simulink library "dxlSimLibrary"  (R2020a)
settings: Solver=VariableStepAuto  StartTime=0.0  StopTime=10.0  RelTol=1e-3
undefined symbols (not defined in the file): group_num_read, group_num_write, lib_name, motor_IDs, motor_models, port_num, protocol_version, select_sync_read, select_sync_write, start_address_read_indirect, Ts
Description:
  | Dynamixel library for Matlab and Simulink
  | Author: Georgios Andrikopoulos (geoand@kth.se), 2022
  | Mechatronics & Embedded Control Systems Unit, KTH, Stockholm
settings Model: Creator=geoand  LastModifiedBy=mluser

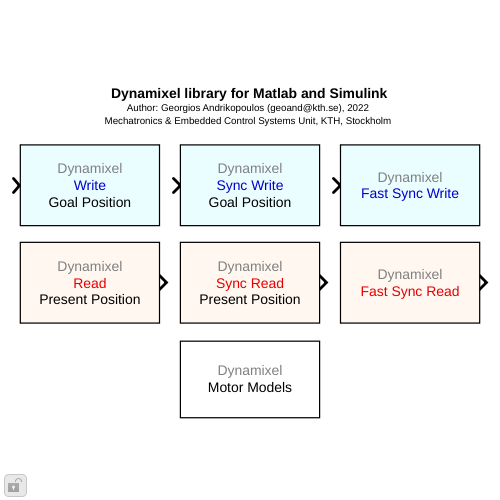
[thumbnail: Simulink's stored preview of the top-level diagram]
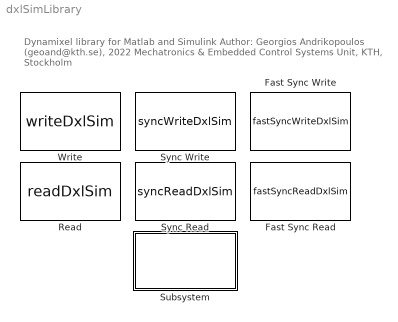
== system dxlSimLibrary ==
  note: Dynamixel library for Matlab and Simulink
      | Author: Georgios Andrikopoulos (geoand@kth.se), 2022
      | Mechatronics & Embedded Control Systems Unit, KTH, Stockholm
  Fast Sync Read : M-S-Function  Description=|  FunctionName=fastSyncReadDxlSim  Parameters=lib_name, group_num_read, ids, models, select_sync_read, start_address_read_indirect, Ts  mask(Dynamixel library for Matlab and Simulink){lib_name=lib_name, group_num_read=group_num_read, ids=motor_IDs, models=motor_models, select_sync_read=select_sync_read, start_address_read_indirect=start_address_read_indirect, Ts=Ts}
      | Dynamixel library for Matlab and Simulink
      | Fast Sync Read function
      | Author: Georgios Andrikopoulos (geoand@kth.se), 2022 
      | Mechatronics & Embedded Control Systems Unit, KTH, Stockholm
      mask prompts: lib_name "Library Name"; group_num_read "Group Number"; ids "Motor IDs"; models "Motor models"; select_sync_read "Sync Read Selection"; start_address_read_indirect "Start Address (Indirect)"; Ts "Sampling Time"
      mask help:
      | Library block for execution of sync read for 1 or more Dynamixel motors in Simulink
      |
      | Part of the Dynamixel library for Matlab and Simulink
      | Author: Georgios Andrikopoulos (geoand@kth.se), 2022
      | Mechatronics & Embedded Control Systems Unit, KTH, Stockholm
      mask Help:
      | Library block for execution of sync read for 1 or more Dynamixel motors in Simulink
      | 
      | Part of the Dynamixel library for Matlab and Simulink
      | Author: Georgios Andrikopoulos (geoand@kth.se), 2022
      | Mechatronics & Embedded Control Systems Unit, KTH, Stockholm
      mask Display:
      | color('gray')
      | fprintf('\nDynamixel\n\n');
      | color('red')
      | fprintf('\n\n\nFast Sync Read\n\n');
  Fast Sync Write : M-S-Function  Description=|  FunctionName=fastSyncWriteDxlSim  Parameters=lib_name, group_num_write, ids, models, select_sync_write, Ts  mask(Dynamixel library for Matlab and Simulink){lib_name=lib_name, group_num_write=group_num_write, ids=motor_IDs, models=motor_models, select_sync_write=select_sync_write, Ts=Ts}
      | Dynamixel library for Matlab and Simulink
      | Fast Sync Write function
      | Author: Georgios Andrikopoulos (geoand@kth.se), 2022 
      | Mechatronics & Embedded Control Systems Unit, KTH, Stockholm
      mask prompts: lib_name "Library Name"; group_num_write "Group Number"; ids "Motor IDs"; models "Motor models"; select_sync_write "Sync Write Parameters"; Ts "Samping Time"
      mask help:
      | Library block for execution of sync write for 1 or more Dynamixel motors in Simulink
      |
      | Part of the Dynamixel library for Matlab and Simulink
      | Author: Georgios Andrikopoulos (geoand@kth.se), 2022
      | Mechatronics & Embedded Control Systems Unit, KTH, Stockholm
      mask Help:
      | Library block for execution of sync write for 1 or more Dynamixel motors in Simulink
      | 
      | Part of the Dynamixel library for Matlab and Simulink
      | Author: Georgios Andrikopoulos (geoand@kth.se), 2022
      | Mechatronics & Embedded Control Systems Unit, KTH, Stockholm
      mask Display:
      | color('gray')
      | fprintf('\nDynamixel\n\n');
      | color('blue')
      | fprintf('\n\n\nFast Sync Write\n\n');
  Read : M-S-Function  Description=|  FunctionName=readDxlSim  Parameters=lib_name, port_num, protocol_version, ids, models, select, Ts  mask(Dynamixel Library for MATLAB and Simulink){lib_name=lib_name, port_num=port_num, protocol_version=protocol_version, ids=motor_IDs, models=motor_models, select=Present Position, Ts=Ts}
      | Dynamixel library for Matlab and Simulink
      | Read function
      | Author: Georgios Andrikopoulos (geoand@kth.se), 2022 
      | Mechatronics & Embedded Control Systems Unit, KTH, Stockholm
      mask prompts: lib_name "Library name"; port_num "Port number"; protocol_version "Protocol version"; ids "Motor IDs"; models "Motor models"; select "Read function"; Ts "Sampling time"
      mask help:
      | Library block executing the read() function for 1 or more Dynamixel motors
      | Part of the Dynamixel library for Matlab and Simulink
      | Author: Georgios Andrikopoulos (geoand@kth.se), 2022
      | Mechatronics & Embedded Control Systems Unit, KTH, Stockholm
      mask Help:
      | Library block executing the read() function for 1 or more Dynamixel motors
      | Part of the Dynamixel library for Matlab and Simulink
      | Author: Georgios Andrikopoulos (geoand@kth.se), 2022
      | Mechatronics & Embedded Control Systems Unit, KTH, Stockholm
      mask Display:
      | color('gray')
      | fprintf('Dynamixel\n\n');
      | color('red')
      | fprintf('\n\nRead\n\n');
      | color('black')
      | fprintf('\n\n%s',select);
  Subsystem : Subsystem  Description=|
      | Dynamixel library for Matlab and Simulink
      | Motor Models
      | Author: Georgios Andrikopoulos (geoand@kth.se), 2022 
      | Mechatronics & Embedded Control Systems Unit, KTH, Stockholm
      mask Display:
      | color('gray')
      | fprintf('Dynamixel\n');
      | color('black')
      | fprintf('\nMotor Models');
  Sync Read : M-S-Function  Description=|  FunctionName=syncReadDxlSim  Parameters=lib_name, group_num, ids, models, select, Ts  mask(Dynamixel Library for MATLAB and Simulink){lib_name=lib_name, group_num=group_num_read(1), ids=motor_IDs, models=motor_models, select=Present Position, Ts=Ts}
      | Dynamixel library for Matlab and Simulink
      | Sync Read function
      | Author: Georgios Andrikopoulos (geoand@kth.se), 2022 
      | Mechatronics & Embedded Control Systems Unit, KTH, Stockholm
      mask prompts: lib_name "Library name"; group_num "Group number"; ids "Motor IDs"; models "Motor models"; select "Read function"; Ts "Sampling time"
      mask help:
      | Library block executing the syncread() function for 1 or more Dynamixel motors
      | Part of the Dynamixel library for Matlab and Simulink
      | Author: Georgios Andrikopoulos (geoand@kth.se), 2022
      | Mechatronics & Embedded Control Systems Unit, KTH, Stockholm
      mask Help:
      | Library block executing the syncread() function for 1 or more Dynamixel motors
      | Part of the Dynamixel library for Matlab and Simulink
      | Author: Georgios Andrikopoulos (geoand@kth.se), 2022
      | Mechatronics & Embedded Control Systems Unit, KTH, Stockholm
      mask Display:
      | color('gray')
      | fprintf('Dynamixel\n\n');
      | color('red')
      | fprintf('\n\nSync Read\n\n');
      | color('black')
      | fprintf('\n\n%s',select);
  Sync Write : M-S-Function  Description=|  FunctionName=syncWriteDxlSim  Parameters=lib_name, group_num, ids, models, select, Ts  mask(Dynamixel Library for MATLAB and Simulink){lib_name=lib_name, group_num=group_num_write(1), ids=motor_IDs, models=motor_models, select=Goal Position, Ts=Ts}
      | Dynamixel library for Matlab and Simulink
      | Sync Write function
      | Author: Georgios Andrikopoulos (geoand@kth.se), 2022 
      | Mechatronics & Embedded Control Systems Unit, KTH, Stockholm
      mask prompts: lib_name "Library name"; group_num "Group number"; ids "Motor IDs"; models "Motor models"; select "Write function"; Ts "Sampling time"
      mask help:
      | Library block executing the syncwrite() function for 1 or more Dynamixel motors
      | Part of the Dynamixel library for Matlab and Simulink
      | Author: Georgios Andrikopoulos (geoand@kth.se), 2022
      | Mechatronics & Embedded Control Systems Unit, KTH, Stockholm
      mask Help:
      | Library block executing the syncwrite() function for 1 or more Dynamixel motors
      | Part of the Dynamixel library for Matlab and Simulink
      | Author: Georgios Andrikopoulos (geoand@kth.se), 2022
      | Mechatronics & Embedded Control Systems Unit, KTH, Stockholm
      mask Display:
      | color('gray')
      | fprintf('Dynamixel\n\n');
      | color('blue')
      | fprintf('\n\nSync Write\n\n');
      | color('black')
      | fprintf('\n\n%s',select);
  Write : M-S-Function  Description=|  FunctionName=writeDxlSim  Parameters=lib_name, port_num, protocol_version, ids, models, select, Ts  mask(Dynamixel Library for MATLAB and Simulink){lib_name=lib_name, port_num=port_num, protocol_version=protocol_version, ids=motor_IDs, models=motor_models, select=Goal Position, Ts=Ts}
      | Dynamixel library for Matlab and Simulink
      | Write function
      | Author: Georgios Andrikopoulos (geoand@kth.se), 2022 
      | Mechatronics & Embedded Control Systems Unit, KTH, Stockholm
      mask prompts: lib_name "Library name"; port_num "Port number"; protocol_version "Protocol version"; ids "Motor IDs"; models "Motor models"; select "Write function"; Ts "Sampling time"
      mask help:
      | Library block executing the write() function for 1 or more Dynamixel motors
      | Part of the Dynamixel library for Matlab and Simulink
      | Author: Georgios Andrikopoulos (geoand@kth.se), 2022
      | Mechatronics & Embedded Control Systems Unit, KTH, Stockholm
      mask Help:
      | Library block executing the write() function for 1 or more Dynamixel motors
      | Part of the Dynamixel library for Matlab and Simulink
      | Author: Georgios Andrikopoulos (geoand@kth.se), 2022
      | Mechatronics & Embedded Control Systems Unit, KTH, Stockholm
      mask Display:
      | color('gray')
      | fprintf('Dynamixel\n\n');
      | color('blue')
      | fprintf('\n\nWrite\n\n');
      | color('black')
      | fprintf('\n\n%s',select);

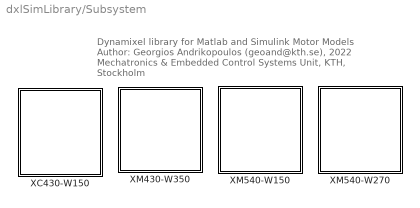
== system dxlSimLibrary/Subsystem ==
  note: Dynamixel library for Matlab and Simulink
      | Motor Models
      | Author: Georgios Andrikopoulos (geoand@kth.se), 2022
      | Mechatronics & Embedded Control Systems Unit, KTH, Stockholm
  XC430-W150 : Subsystem  Description=|
      | Dynamixel library for Matlab and Simulink
      | Motor Models
      | Author: Georgios Andrikopoulos (geoand@kth.se), 2022 
      | Mechatronics & Embedded Control Systems Unit, KTH, Stockholm
      mask Display: image('$imagefile'); % Use "Edit Image" on toolstrip to change.
  "XM430-W350 " : Subsystem  Description=|
      | Dynamixel library for Matlab and Simulink
      | Motor Models
      | Author: Georgios Andrikopoulos (geoand@kth.se), 2022 
      | Mechatronics & Embedded Control Systems Unit, KTH, Stockholm
      mask Display: image('$imagefile'); % Use "Edit Image" on toolstrip to change.
  XM540-W150 : Subsystem  Description=|
      | Dynamixel library for Matlab and Simulink
      | Motor Models
      | Author: Georgios Andrikopoulos (geoand@kth.se), 2022 
      | Mechatronics & Embedded Control Systems Unit, KTH, Stockholm
      mask Display: image('$imagefile'); % Use "Edit Image" on toolstrip to change.
  XM540-W270 : Subsystem  Description=|
      | Dynamixel library for Matlab and Simulink
      | Motor Models
      | Author: Georgios Andrikopoulos (geoand@kth.se), 2022 
      | Mechatronics & Embedded Control Systems Unit, KTH, Stockholm
      mask Display: image('$imagefile'); % Use "Edit Image" on toolstrip to change.

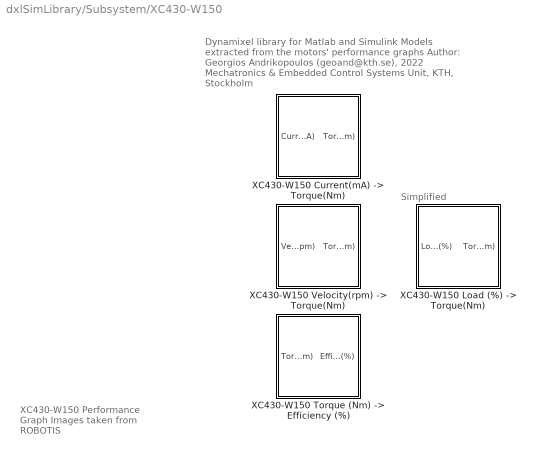
== system dxlSimLibrary/Subsystem/XC430-W150 ==
  note: Simplified
  note: Dynamixel library for Matlab and Simulink
      | Models extracted from the motors' performance graphs
      | Author: Georgios Andrikopoulos (geoand@kth.se), 2022
      | Mechatronics & Embedded Control Systems Unit, KTH, Stockholm
  note: XC430-W150 Performance Graph
      | Images taken from ROBOTIS
  "XC430-W150 Current(mA) -> Torque(Nm)" : Subsystem  Description=|
      | Dynamixel library for Matlab and Simulink
      | Author: Georgios Andrikopoulos (geoand@kth.se), 2022 
      | Mechatronics & Embedded Control Systems Unit, KTH, Stockholm
      mask Display: image('$imagefile'); % Use "Edit Image" on toolstrip to change.
  "XC430-W150 Load (%) -> Torque(Nm)" : Subsystem  Description=|
      | Dynamixel library for Matlab and Simulink
      | Author: Georgios Andrikopoulos (geoand@kth.se), 2022 
      | Mechatronics & Embedded Control Systems Unit, KTH, Stockholm
      mask Display: image('$imagefile'); % Use "Edit Image" on toolstrip to change.
  "XC430-W150 Torque (Nm) -> Efficiency (%)" : Subsystem  Description=|
      | Dynamixel library for Matlab and Simulink
      | Author: Georgios Andrikopoulos (geoand@kth.se), 2022 
      | Mechatronics & Embedded Control Systems Unit, KTH, Stockholm
      mask Display: image('$imagefile'); % Use "Edit Image" on toolstrip to change.
  "XC430-W150 Velocity(rpm) -> Torque(Nm)" : Subsystem  Description=|
      | Dynamixel library for Matlab and Simulink
      | Author: Georgios Andrikopoulos (geoand@kth.se), 2022 
      | Mechatronics & Embedded Control Systems Unit, KTH, Stockholm
      mask Display: image('$imagefile'); % Use "Edit Image" on toolstrip to change.

== system dxlSimLibrary/Subsystem/XM430-W350  ==
  note: Dynamixel library for Matlab and Simulink
      | Models extracted from the motors' performance graphs
      | Author: Georgios Andrikopoulos (geoand@kth.se), 2022
      | Mechatronics & Embedded Control Systems Unit, KTH, Stockholm
  note: XM430-W350 Performance Graph
      | Images taken from ROBOTIS
  "XM430-W350 Current(mA) -> Torque(Nm)" : Subsystem  Description=|
      | Dynamixel library for Matlab and Simulink
      | Author: Georgios Andrikopoulos (geoand@kth.se), 2022 
      | Mechatronics & Embedded Control Systems Unit, KTH, Stockholm
      mask Display: image('$imagefile'); % Use "Edit Image" on toolstrip to change.
  "XM430-W350 Torque (Nm) -> Efficiency (%)" : Subsystem  Description=|
      | Dynamixel library for Matlab and Simulink
      | Author: Georgios Andrikopoulos (geoand@kth.se), 2022 
      | Mechatronics & Embedded Control Systems Unit, KTH, Stockholm
      mask Display: image('$imagefile'); % Use "Edit Image" on toolstrip to change.
  "XM430-W350 Velocity(rpm) -> Torque(Nm)" : Subsystem  Description=|
      | Dynamixel library for Matlab and Simulink
      | Author: Georgios Andrikopoulos (geoand@kth.se), 2022 
      | Mechatronics & Embedded Control Systems Unit, KTH, Stockholm
      mask Display: image('$imagefile'); % Use "Edit Image" on toolstrip to change.

== system dxlSimLibrary/Subsystem/XM540-W150 ==
  note: Dynamixel library for Matlab and Simulink
      | Models extracted from the motors' performance graphs
      | Author: Georgios Andrikopoulos (geoand@kth.se), 2022
      | Mechatronics & Embedded Control Systems Unit, KTH, Stockholm
  note: XM540-W150 Performance Graph
      | Images taken from ROBOTIS
  "XM540-W150 Current(mA) -> Torque(Nm)" : Subsystem  Description=|
      | Dynamixel library for Matlab and Simulink
      | Author: Georgios Andrikopoulos (geoand@kth.se), 2022 
      | Mechatronics & Embedded Control Systems Unit, KTH, Stockholm
      mask Display: image('$imagefile'); % Use "Edit Image" on toolstrip to change.
  "XM540-W150 Torque (Nm) -> Efficiency (%)" : Subsystem  Description=|
      | Dynamixel library for Matlab and Simulink
      | Author: Georgios Andrikopoulos (geoand@kth.se), 2022 
      | Mechatronics & Embedded Control Systems Unit, KTH, Stockholm
      mask Display: image('$imagefile'); % Use "Edit Image" on toolstrip to change.
  "XM540-W150 Velocity(rpm) -> Torque(Nm)" : Subsystem  Description=|
      | Dynamixel library for Matlab and Simulink
      | Author: Georgios Andrikopoulos (geoand@kth.se), 2022 
      | Mechatronics & Embedded Control Systems Unit, KTH, Stockholm
      mask Display: image('$imagefile'); % Use "Edit Image" on toolstrip to change.

== system dxlSimLibrary/Subsystem/XM540-W270 ==
  note: Dynamixel library for Matlab and Simulink
      | Models extracted from the motors' performance graphs
      | Author: Georgios Andrikopoulos (geoand@kth.se), 2022
      | Mechatronics & Embedded Control Systems Unit, KTH, Stockholm
  note: XM540-W270 Performance Graph
      | Images taken from ROBOTIS
  "XM540-W270 Current(mA) -> Torque(Nm)" : Subsystem  Description=|
      | Dynamixel library for Matlab and Simulink
      | Author: Georgios Andrikopoulos (geoand@kth.se), 2022 
      | Mechatronics & Embedded Control Systems Unit, KTH, Stockholm
      mask Display: image('$imagefile'); % Use "Edit Image" on toolstrip to change.
  "XM540-W270 Torque (Nm) -> Efficiency (%)" : Subsystem  Description=|
      | Dynamixel library for Matlab and Simulink
      | Author: Georgios Andrikopoulos (geoand@kth.se), 2022 
      | Mechatronics & Embedded Control Systems Unit, KTH, Stockholm
      mask Display: image('$imagefile'); % Use "Edit Image" on toolstrip to change.
  "XM540-W270 Velocity(rpm) -> Torque(Nm)" : Subsystem  Description=|
      | Dynamixel library for Matlab and Simulink
      | Author: Georgios Andrikopoulos (geoand@kth.se), 2022 
      | Mechatronics & Embedded Control Systems Unit, KTH, Stockholm
      mask Display: image('$imagefile'); % Use "Edit Image" on toolstrip to change.

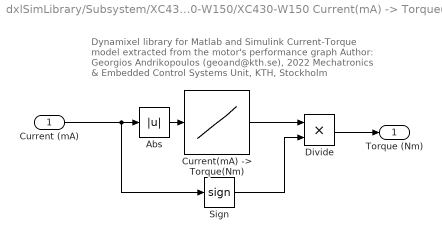
== system dxlSimLibrary/Subsystem/XC430-W150/XC430-W150 Current(mA) -> Torque(Nm) ==
  note: Dynamixel library for Matlab and Simulink
      | Current-Torque model extracted from the motor's performance graph
      | Author: Georgios Andrikopoulos (geoand@kth.se), 2022
      | Mechatronics & Embedded Control Systems Unit, KTH, Stockholm
  Current (mA) : Inport
  Abs : Abs
  "Current(mA) -> Torque(Nm)" : Lookup_n-D  NumberOfTableDimensions=1  BreakpointsForDimension1="[0 200    218    334    458    602    766    952    1164    1270]"  BreakpointsForDimension1DataTypeStr=double  Table="[0 0.0890    0.1030    0.2000    0.3000    0.4000    0.5000    0.6000    0.7000    0.7420]"  TableDataTypeStr=double  IntermediateResultsDataTypeStr=double  InternalRulePriority=Speed  OutDataTypeStr=double  RndMeth=Simplest  FractionDataTypeStr=double
  Divide : Product  Inputs=**
  Sign : Signum
  Torque (Nm) : Outport
  wires:
  Abs/1 -> "Current(mA) -> Torque(Nm)"/1
  "Current(mA) -> Torque(Nm)"/1 -> Divide/1
  Divide/1 -> Torque (Nm)/1
  Sign/1 -> Divide/2
  Current (mA)/1 -> Sign/1, Abs/1

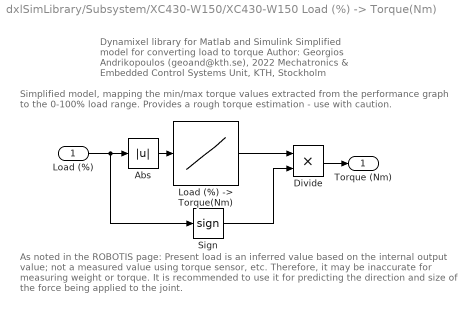
== system dxlSimLibrary/Subsystem/XC430-W150/XC430-W150 Load (%) -> Torque(Nm) ==
  note: As noted in the ROBOTIS page:
      | Present load is an inferred value based on the internal output value; not a measured value using torque sensor, etc. Therefore, it may be inaccurate for measuring weight or torque. It is recommended to use it for predicting the direction and size of the force being applied to the joint.
  note: Simplified model, mapping the min/max torque values extracted from the performance graph to the 0-100% load range. Provides a rough torque estimation - use with caution.
  note: Dynamixel library for Matlab and Simulink
      | Simplified model for converting load to torque
      | Author: Georgios Andrikopoulos (geoand@kth.se), 2022
      | Mechatronics & Embedded Control Systems Unit, KTH, Stockholm
  Load (%) : Inport
  Abs : Abs
  Divide : Product  Inputs=**
  "Load (%) -> Torque(Nm)" : Lookup_n-D  NumberOfTableDimensions=1  BreakpointsForDimension1=[0 100]  BreakpointsForDimension1DataTypeStr=double  Table=[0.0890 0.7420]  TableDataTypeStr=double  IntermediateResultsDataTypeStr=double  InternalRulePriority=Speed  OutDataTypeStr=double  RndMeth=Simplest  FractionDataTypeStr=double
  Sign : Signum
  Torque (Nm) : Outport
  wires:
  Load (%)/1 -> Sign/1, Abs/1
  "Load (%) -> Torque(Nm)"/1 -> Divide/1
  Abs/1 -> "Load (%) -> Torque(Nm)"/1
  Sign/1 -> Divide/2
  Divide/1 -> Torque (Nm)/1

== system dxlSimLibrary/Subsystem/XC430-W150/XC430-W150 Torque (Nm) -> Efficiency (%) ==
  note: Dynamixel library for Matlab and Simulink
      | Torque-Efficiency model extracted from the motor's performance graph
      | Author: Georgios Andrikopoulos (geoand@kth.se), 2022
      | Mechatronics & Embedded Control Systems Unit, KTH, Stockholm
  Torque (Nm) : Inport
  Abs1 : Abs
  "Torque (Nm) -> Efficiency (%)" : Lookup_n-D  NumberOfTableDimensions=1  BreakpointsForDimension1="[0.0890    0.1030    0.2000    0.3000    0.4000    0.5000    0.6000    0.7000    0.7420]"  BreakpointsForDimension1DataTypeStr=Inherit: Inherit from 'Breakpoint data'  Table="[36.7000   40.0000   46.1000   43.3000   37.9000   31.0000   21.6000   10.5000    5.2000]"  InternalRulePriority=Speed  RndMeth=Simplest  InputSameDT=on
  Efficiency (%) : Outport
  wires:
  "Torque (Nm) -> Efficiency (%)"/1 -> Efficiency (%)/1
  Abs1/1 -> "Torque (Nm) -> Efficiency (%)"/1
  Torque (Nm)/1 -> Abs1/1

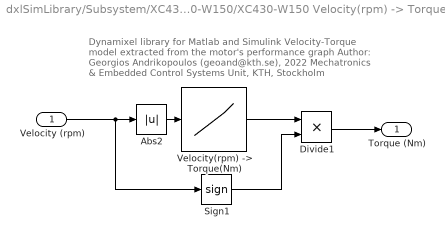
== system dxlSimLibrary/Subsystem/XC430-W150/XC430-W150 Velocity(rpm) -> Torque(Nm) ==
  note: Dynamixel library for Matlab and Simulink
      | Velocity-Torque model extracted from the motor's performance graph
      | Author: Georgios Andrikopoulos (geoand@kth.se), 2022
      | Mechatronics & Embedded Control Systems Unit, KTH, Stockholm
  Velocity (rpm) : Inport
  Abs2 : Abs
  Divide1 : Product  Inputs=**
  Sign1 : Signum
  "Velocity(rpm) -> Torque(Nm)" : Lookup_n-D  NumberOfTableDimensions=1  BreakpointsForDimension1="[7.7000   18.0400   37.4000   53.4600   67.1000   78.9800   89.4300   98.7800  100.2100]"  BreakpointsForDimension1DataTypeStr=double  Table="[0.7420    0.7000    0.6000    0.5000    0.4000    0.3000    0.2000    0.1030    0.0890]"  TableDataTypeStr=double  IntermediateResultsDataTypeStr=double  InternalRulePriority=Speed  OutDataTypeStr=double  RndMeth=Simplest  FractionDataTypeStr=double  InputSameDT=on
  Torque (Nm) : Outport
  wires:
  Divide1/1 -> Torque (Nm)/1
  Velocity (rpm)/1 -> Sign1/1, Abs2/1
  Sign1/1 -> Divide1/2
  Abs2/1 -> "Velocity(rpm) -> Torque(Nm)"/1
  "Velocity(rpm) -> Torque(Nm)"/1 -> Divide1/1

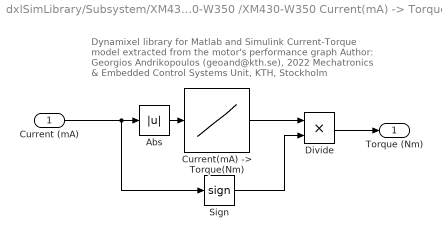
== system dxlSimLibrary/Subsystem/XM430-W350 /XM430-W350 Current(mA) -> Torque(Nm) ==
  note: Dynamixel library for Matlab and Simulink
      | Current-Torque model extracted from the motor's performance graph
      | Author: Georgios Andrikopoulos (geoand@kth.se), 2022
      | Mechatronics & Embedded Control Systems Unit, KTH, Stockholm
  Current (mA) : Inport
  Abs : Abs
  "Current(mA) -> Torque(Nm)" : Lookup_n-D  NumberOfTableDimensions=1  BreakpointsForDimension1=|  BreakpointsForDimension1DataTypeStr=double  Table=|  TableDataTypeStr=double  IntermediateResultsDataTypeStr=double  InternalRulePriority=Speed  OutDataTypeStr=double  RndMeth=Simplest  FractionDataTypeStr=double
      BreakpointsForDimension1=|
      | [0; 114
      | 270
      | 471
      | 672
      | 867
      | 1080
      | 1275
      | 1485
      | 1692
      | 1797]
      Table=|
      | [0; 0.056
      | 0.350
      | 0.700
      | 1.050
      | 1.400
      | 1.750
      | 2.100
      | 2.450
      | 2.800
      | 3.010]
  Divide : Product  Inputs=**
  Sign : Signum
  Torque (Nm) : Outport
  wires:
  Abs/1 -> "Current(mA) -> Torque(Nm)"/1
  "Current(mA) -> Torque(Nm)"/1 -> Divide/1
  Divide/1 -> Torque (Nm)/1
  Sign/1 -> Divide/2
  Current (mA)/1 -> Sign/1, Abs/1

== system dxlSimLibrary/Subsystem/XM430-W350 /XM430-W350 Torque (Nm) -> Efficiency (%) ==
  note: Dynamixel library for Matlab and Simulink
      | Torque-Efficiency model extracted from the motor's performance graph
      | Author: Georgios Andrikopoulos (geoand@kth.se), 2022
      | Mechatronics & Embedded Control Systems Unit, KTH, Stockholm
  Current (mA) : Inport
  Abs1 : Abs
  "Torque (Nm) -> Efficiency (%)" : Lookup_n-D  NumberOfTableDimensions=1  BreakpointsForDimension1=[0.056,0.350,0.700,1.050,1.400,1.750,2.100,2.450,2.800,3.010]  BreakpointsForDimension1DataTypeStr=Inherit: Inherit from 'Breakpoint data'  Table=[12.70,35,43.50,44.30,41.20,36,29.70,22.40,14.50,9.70]  InternalRulePriority=Speed  RndMeth=Simplest  InputSameDT=on
  Torque (Nm) : Outport
  wires:
  Abs1/1 -> "Torque (Nm) -> Efficiency (%)"/1
  "Torque (Nm) -> Efficiency (%)"/1 -> Torque (Nm)/1
  Current (mA)/1 -> Abs1/1

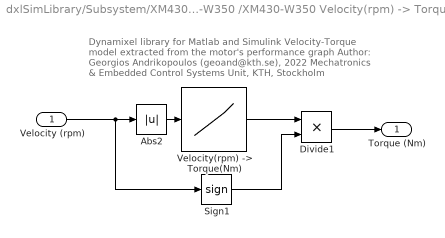
== system dxlSimLibrary/Subsystem/XM430-W350 /XM430-W350 Velocity(rpm) -> Torque(Nm) ==
  note: Dynamixel library for Matlab and Simulink
      | Velocity-Torque model extracted from the motor's performance graph
      | Author: Georgios Andrikopoulos (geoand@kth.se), 2022
      | Mechatronics & Embedded Control Systems Unit, KTH, Stockholm
  Velocity (rpm) : Inport
  Abs2 : Abs
  Divide1 : Product  Inputs=**
  Sign1 : Signum
  "Velocity(rpm) -> Torque(Nm)" : Lookup_n-D  NumberOfTableDimensions=1  BreakpointsForDimension1=[7.76,10.32,14.96,19.60,24,28.56,33.04,37.68,42.08,46.08]  BreakpointsForDimension1DataTypeStr=double  Table=[3.010,2.800,2.450,2.100,1.750,1.400,1.050,0.700,0.350,0.056]  TableDataTypeStr=double  IntermediateResultsDataTypeStr=double  InternalRulePriority=Speed  OutDataTypeStr=double  RndMeth=Simplest  FractionDataTypeStr=double  InputSameDT=on
  Torque (Nm) : Outport
  wires:
  Sign1/1 -> Divide1/2
  Divide1/1 -> Torque (Nm)/1
  Velocity (rpm)/1 -> Sign1/1, Abs2/1
  "Velocity(rpm) -> Torque(Nm)"/1 -> Divide1/1
  Abs2/1 -> "Velocity(rpm) -> Torque(Nm)"/1

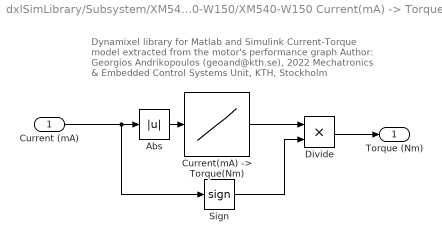
== system dxlSimLibrary/Subsystem/XM540-W150/XM540-W150 Current(mA) -> Torque(Nm) ==
  note: Dynamixel library for Matlab and Simulink
      | Current-Torque model extracted from the motor's performance graph
      | Author: Georgios Andrikopoulos (geoand@kth.se), 2022
      | Mechatronics & Embedded Control Systems Unit, KTH, Stockholm
  Current (mA) : Inport
  Abs : Abs
  "Current(mA) -> Torque(Nm)" : Lookup_n-D  NumberOfTableDimensions=1  BreakpointsForDimension1=|  BreakpointsForDimension1DataTypeStr=double  Table=[0 0.4 0.5 1 1.5 2 2.5 3 3.5 4 4.5]  TableDataTypeStr=double  IntermediateResultsDataTypeStr=double  InternalRulePriority=Speed  OutDataTypeStr=double  RndMeth=Simplest  FractionDataTypeStr=double
      | [0 546
      | 623
      | 1050
      | 1477
      | 1953
      | 2429
      | 2933
      | 3486
      | 4067
      | 4683]
  Divide : Product  Inputs=**
  Sign : Signum
  Torque (Nm) : Outport
  wires:
  Abs/1 -> "Current(mA) -> Torque(Nm)"/1
  "Current(mA) -> Torque(Nm)"/1 -> Divide/1
  Divide/1 -> Torque (Nm)/1
  Sign/1 -> Divide/2
  Current (mA)/1 -> Sign/1, Abs/1

== system dxlSimLibrary/Subsystem/XM540-W150/XM540-W150 Torque (Nm) -> Efficiency (%) ==
  note: Dynamixel library for Matlab and Simulink
      | Torque-Efficiency model extracted from the motor's performance graph
      | Author: Georgios Andrikopoulos (geoand@kth.se), 2022
      | Mechatronics & Embedded Control Systems Unit, KTH, Stockholm
  Current (mA) : Inport
  Abs1 : Abs
  "Torque (Nm) -> Efficiency (%)" : Lookup_n-D  NumberOfTableDimensions=1  BreakpointsForDimension1=[0.4 0.5 1 1.5 2 2.5 3 3.5 4 4.5]  BreakpointsForDimension1DataTypeStr=Inherit: Inherit from 'Breakpoint data'  Table=|  InternalRulePriority=Speed  RndMeth=Simplest  InputSameDT=on
      | [   34.9000
      |    40.0000
      |    49.5000
      |    49.7000
      |    44.8000
      |    38.2000
      |    30.4000
      |    22.0000
      |    13.1000
      |     3.8000]
  Torque (Nm) : Outport
  wires:
  Abs1/1 -> "Torque (Nm) -> Efficiency (%)"/1
  "Torque (Nm) -> Efficiency (%)"/1 -> Torque (Nm)/1
  Current (mA)/1 -> Abs1/1

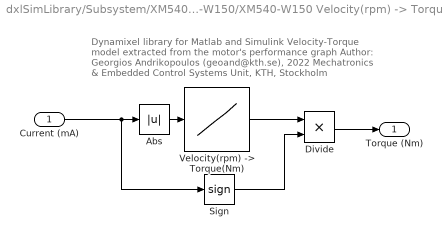
== system dxlSimLibrary/Subsystem/XM540-W150/XM540-W150 Velocity(rpm) -> Torque(Nm) ==
  note: Dynamixel library for Matlab and Simulink
      | Velocity-Torque model extracted from the motor's performance graph
      | Author: Georgios Andrikopoulos (geoand@kth.se), 2022
      | Mechatronics & Embedded Control Systems Unit, KTH, Stockholm
  Current (mA) : Inport
  Abs : Abs
  Divide : Product  Inputs=**
  Sign : Signum
  "Velocity(rpm) -> Torque(Nm)" : Lookup_n-D  NumberOfTableDimensions=1  BreakpointsForDimension1=|  BreakpointsForDimension1DataTypeStr=double  Table=[4.5 4 3.5 3 2.5 2 1.5 1 0.5 0.4]  TableDataTypeStr=double  IntermediateResultsDataTypeStr=double  InternalRulePriority=Speed  OutDataTypeStr=double  RndMeth=Simplest  FractionDataTypeStr=double  InputSameDT=on
      | [    4.4800
      |    13.3700
      |    21.5600
      |    29.4700
      |    36.6800
      |    43.5400
      |    50.4000
      |    56.7000
      |    63.0000
      |    64.1200]
  Torque (Nm) : Outport
  wires:
  Abs/1 -> "Velocity(rpm) -> Torque(Nm)"/1
  "Velocity(rpm) -> Torque(Nm)"/1 -> Divide/1
  Divide/1 -> Torque (Nm)/1
  Sign/1 -> Divide/2
  Current (mA)/1 -> Sign/1, Abs/1

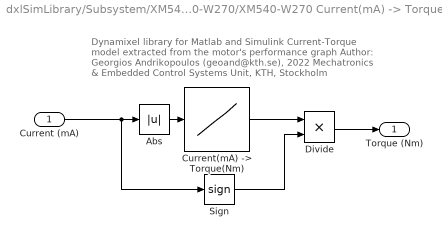
== system dxlSimLibrary/Subsystem/XM540-W270/XM540-W270 Current(mA) -> Torque(Nm) ==
  note: Dynamixel library for Matlab and Simulink
      | Current-Torque model extracted from the motor's performance graph
      | Author: Georgios Andrikopoulos (geoand@kth.se), 2022
      | Mechatronics & Embedded Control Systems Unit, KTH, Stockholm
  Current (mA) : Inport
  Abs : Abs
  "Current(mA) -> Torque(Nm)" : Lookup_n-D  NumberOfTableDimensions=1  BreakpointsForDimension1=|  BreakpointsForDimension1DataTypeStr=double  Table=|  TableDataTypeStr=double  IntermediateResultsDataTypeStr=double  InternalRulePriority=Speed  OutDataTypeStr=double  RndMeth=Simplest  FractionDataTypeStr=double
      BreakpointsForDimension1=|
      | [0; 301
      | 497
      | 847
      | 1246
      | 1659
      | 2114
      | 2597
      | 3129
      | 3703
      | 4060]
      Table=|
      | [0; 0.4
      | 1
      | 2
      | 3
      | 4
      | 5
      | 6
      | 7
      | 8
      | 8.6]
  Divide : Product  Inputs=**
  Sign : Signum
  Torque (Nm) : Outport
  wires:
  Abs/1 -> "Current(mA) -> Torque(Nm)"/1
  "Current(mA) -> Torque(Nm)"/1 -> Divide/1
  Divide/1 -> Torque (Nm)/1
  Sign/1 -> Divide/2
  Current (mA)/1 -> Sign/1, Abs/1

== system dxlSimLibrary/Subsystem/XM540-W270/XM540-W270 Torque (Nm) -> Efficiency (%) ==
  note: Dynamixel library for Matlab and Simulink
      | Torque-Efficiency model extracted from the motor's performance graph
      | Author: Georgios Andrikopoulos (geoand@kth.se), 2022
      | Mechatronics & Embedded Control Systems Unit, KTH, Stockholm
  Current (mA) : Inport
  Abs1 : Abs
  "Torque(Nm) -> Efficiency(%)" : Lookup_n-D  NumberOfTableDimensions=1  BreakpointsForDimension1=|  BreakpointsForDimension1DataTypeStr=Inherit: Inherit from 'Breakpoint data'  Table=|  InternalRulePriority=Speed  RndMeth=Simplest  InputSameDT=on
      BreakpointsForDimension1=|
      | [0.4
      | 1
      | 2
      | 3
      | 4
      | 5
      | 6
      | 7
      | 8
      | 8.6]
      Table=|
      | [28.2
      | 40
      | 46
      | 44.4
      | 40
      | 34.6
      | 28.1
      | 20.7
      | 11.7
      | 5.2]
  Torque (Nm) : Outport
  wires:
  Abs1/1 -> "Torque(Nm) -> Efficiency(%)"/1
  "Torque(Nm) -> Efficiency(%)"/1 -> Torque (Nm)/1
  Current (mA)/1 -> Abs1/1

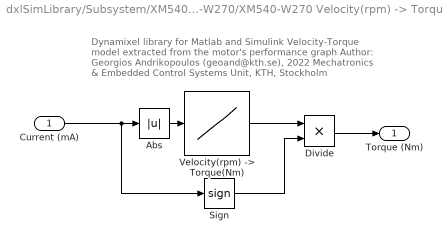
== system dxlSimLibrary/Subsystem/XM540-W270/XM540-W270 Velocity(rpm) -> Torque(Nm) ==
  note: Dynamixel library for Matlab and Simulink
      | Velocity-Torque model extracted from the motor's performance graph
      | Author: Georgios Andrikopoulos (geoand@kth.se), 2022
      | Mechatronics & Embedded Control Systems Unit, KTH, Stockholm
  Current (mA) : Inport
  Abs : Abs
  Divide : Product  Inputs=**
  Sign : Signum
  "Velocity(rpm) -> Torque(Nm)" : Lookup_n-D  NumberOfTableDimensions=1  BreakpointsForDimension1=[2.100000000000000;4.935000000000000;9.030000000000000;12.635000000000000;15.925000000000000;19.040000000000000;21.910000000000000;24.675000000000000;27.335000000000000;28.875000000000000]  BreakpointsForDimension1DataTypeStr=double  Table=[8.6,8,7,6,5,4,3,2,1,0.4]  TableDataTypeStr=double  IntermediateResultsDataTypeStr=double  InternalRulePriority=Speed  OutDataTypeStr=double  RndMeth=Simplest  FractionDataTypeStr=double  InputSameDT=on
  Torque (Nm) : Outport
  wires:
  Abs/1 -> "Velocity(rpm) -> Torque(Nm)"/1
  "Velocity(rpm) -> Torque(Nm)"/1 -> Divide/1
  Divide/1 -> Torque (Nm)/1
  Sign/1 -> Divide/2
  Current (mA)/1 -> Sign/1, Abs/1
